simulink model "Coomputation_Cov"  (R2016b)
settings: Solver=VariableStepAuto  StartTime=0.0  StopTime=10.0  RelTol=1e-3
settings Model: Creator=liana  LastModifiedBy=liana

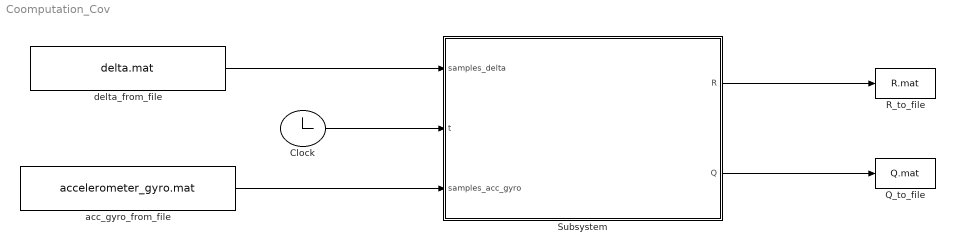
== system Coomputation_Cov ==
  Clock : Clock
      settings: Decimation=100
  Q_to_file : ToFile  Filename=Q.mat  SaveFormat=Timeseries
  R_to_file : ToFile  Filename=R.mat  SaveFormat=Timeseries
  Subsystem : Subsystem
  acc_gyro_from_file : FromFile  FileName=accelerometer_gyro.mat  SampleTime=0
  delta_from_file : FromFile  FileName=delta.mat  SampleTime=0
  wires:
  delta_from_file/1 -> Subsystem/1(samples_delta)
  Clock/1 -> Subsystem/2(t)
  acc_gyro_from_file/1 -> Subsystem/3(samples_acc_gyro)
  Subsystem/1(R) -> R_to_file/1
  Subsystem/2(Q) -> Q_to_file/1

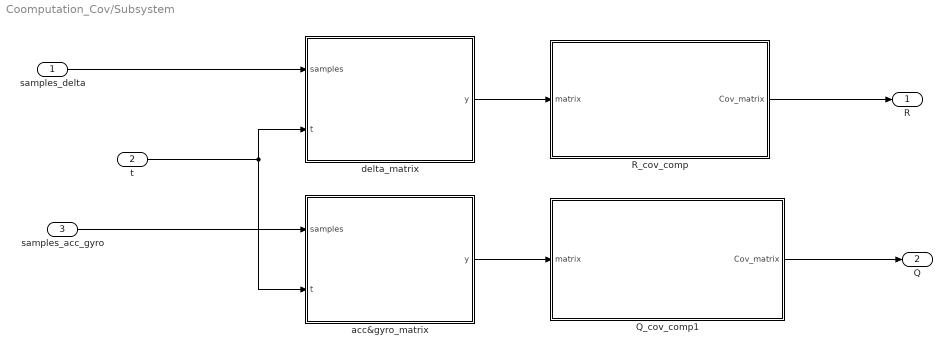
== system Coomputation_Cov/Subsystem ==
  samples_delta : Inport
  t : Inport  Port=2
  samples_acc_gyro : Inport  Port=3
  Q_cov_comp1 : MATLAB Function  TreatAsAtomicUnit=on
  R_cov_comp : MATLAB Function  TreatAsAtomicUnit=on
  acc&gyro_matrix : MATLAB Function  TreatAsAtomicUnit=on
  delta_matrix : MATLAB Function  TreatAsAtomicUnit=on
  R : Outport
  Q : Outport  Port=2
  wires:
  acc&gyro_matrix/1(y) -> Q_cov_comp1/1(matrix)
  R_cov_comp/1(Cov_matrix) -> R/1
  t/1 -> acc&gyro_matrix/2(t), delta_matrix/2(t)
  Q_cov_comp1/1(Cov_matrix) -> Q/1
  delta_matrix/1(y) -> R_cov_comp/1(matrix)
  samples_acc_gyro/1 -> acc&gyro_matrix/1(samples)
  samples_delta/1 -> delta_matrix/1(samples)

== matlab function Coomputation_Cov/Subsystem/Q_cov_comp1 ==
  data: matrix input; Cov_matrix output
function Cov_matrix = covariance_comp(matrix)

 % m - rows equal to the number of measures of the variables
 % n - cols equal to the number of samples
    
row = size(matrix,1);

Cov_matrix = zeros(row);

for i = 1:1:row
    
   Cov_matrix(i,i) = cov(matrix(i,:));
    
end

Cov_matrix;


% to make a simulink block for initialization

== matlab function Coomputation_Cov/Subsystem/delta_matrix ==
  data: samples input; y output; t input
function y = building_delta(samples, t)

row = size(samples,1);

if t == 0
    % the initialisation window counts 100 samples
    matrix = zeros(row, 100);
end

matrix(:,t) = samples;

if t == 100
    % the output should be sent when the last sample comes
    y = matrix;
end



%
% matrix = [];
%
% matrix = [ matrix samples] ;
%

== matlab function Coomputation_Cov/Subsystem/acc&gyro_matrix ==
  data: samples input; y output; t input
function y = building_acc_gyro(samples, t)

row = size(samples,1);

if t == 0
    % the initialisation window counts 100 samples
    matrix = zeros(row, 100);
end

matrix(:,t) = samples;

if t == 100
    % the output should be sent when the last sample comes
    y = matrix;
end

== matlab function Coomputation_Cov/Subsystem/R_cov_comp ==
  data: matrix input; Cov_matrix output
function Cov_matrix = covariance_comp(matrix)

 % m - rows equal to the number of measures of the variables
 % n - cols equal to the number of samples
    
row = size(matrix,1);

Cov_matrix = zeros(row);

for i = 1:1:row
    
   Cov_matrix(i,i) = cov(matrix(i,:));
    
end

Cov_matrix;


% to make a simulink block for initialization
